simulink model "drei_b"  (R2023a)
settings: Solver=VariableStepAuto  StartTime=0.0  StopTime=10.0  RelTol=1e-3
settings Model: Creator=alexa  LastModifiedBy=alexa

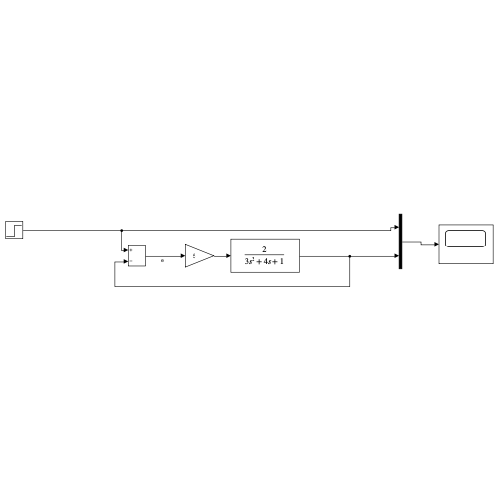
[thumbnail: Simulink's stored preview of the top-level diagram]
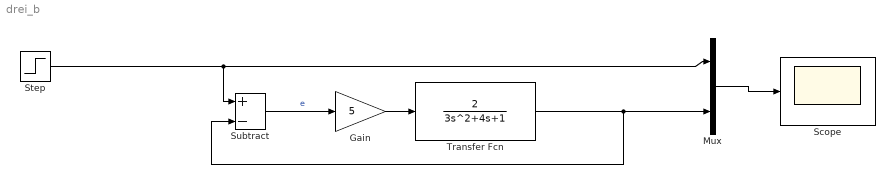
== system drei_b ==
  Gain : Gain  Gain=5
  Mux : Mux  Inputs=2
  Scope : Scope
  Step : Step  SampleTime=0
  Subtract : Sum  Inputs=+-
  Transfer Fcn : TransferFcn  Numerator=[2]  Denominator=[3 4 1]
  wires:
  Step/1 -> Subtract/1, Mux/1
  Subtract/1 -> Gain/1  "e"
  Gain/1 -> Transfer Fcn/1
  Transfer Fcn/1 -> Subtract/2, Mux/2
  Mux/1 -> Scope/1
